simulink model "svpwm_inv_ideal_switch_Motor_new"  (R2025a)
settings: Solver=daessc  StartTime=0.0  StopTime=0.5  MaxStep=1e-7  RelTol=1e-3
undefined symbols (not defined in the file): Down, Up
libraries: fl_lib x20, nesl_utility x19, ee_lib x14, mcbeeMathTransformLib x7, slpidlib x4, eePwmGenerator x3, spsMeanLib x2, simulink_extras x1
(part 2 of 2)

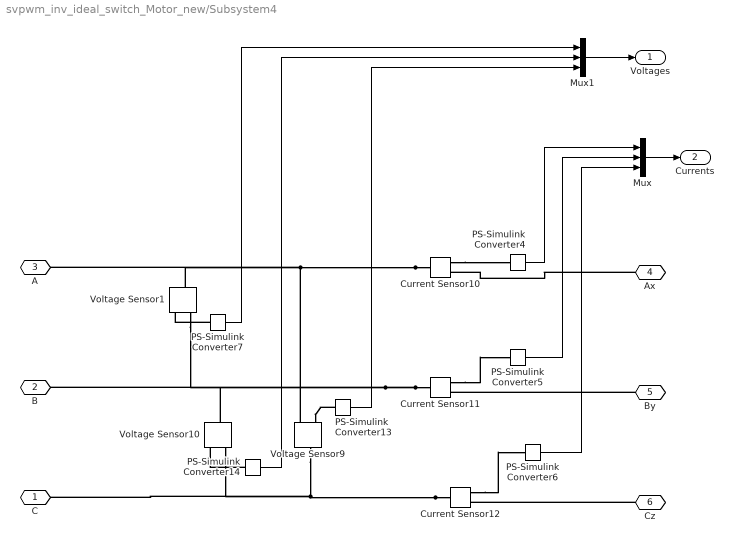
== system svpwm_inv_ideal_switch_Motor_new/Subsystem4 ==
  Current Sensor10 : fl_lib/Electrical/Electrical Sensors/Current Sensor
  Current Sensor11 : fl_lib/Electrical/Electrical Sensors/Current Sensor
  Current Sensor12 : fl_lib/Electrical/Electrical Sensors/Current Sensor
  Mux : Mux  Inputs=3
  Mux1 : Mux  Inputs=3
  PS-Simulink Converter{4..7,13..14} (6 alike) : nesl_utility/PS-Simulink Converter  PhysicalDomain=network_engine_domain  SubClassName=ps_output  LeftPortType=input  RightPortType=output  PseudoPeriodic=off  Frequencies=[]  VectorFormat=inherit  Unit=inherit  AffineConversion=off
  Voltage Sensor1 : fl_lib/Electrical/Electrical Sensors/Voltage Sensor
  Voltage Sensor10 : fl_lib/Electrical/Electrical Sensors/Voltage Sensor
  Voltage Sensor9 : fl_lib/Electrical/Electrical Sensors/Voltage Sensor
  C : PMIOPort  Side=Left
  B : PMIOPort  Port=2  Side=Left
  A : PMIOPort  Port=3  Side=Left
  Ax : PMIOPort  Port=4  Side=Right
  By : PMIOPort  Port=5  Side=Right
  Cz : PMIOPort  Port=6  Side=Right
  Voltages : Outport
  Currents : Outport  Port=2
  wires:
  Mux1/1 -> Voltages/1
  Mux/1 -> Currents/1
  PS-Simulink Converter7/1 -> Mux1/1
  PS-Simulink Converter14/1 -> Mux1/2
  PS-Simulink Converter4/1 -> Mux/1
  PS-Simulink Converter13/1 -> Mux1/3
  PS-Simulink Converter6/1 -> Mux/3
  PS-Simulink Converter5/1 -> Mux/2
  connections:
  By/RConn1 -- Current Sensor11/RConn2
  PS-Simulink Converter7/LConn1 -- Voltage Sensor1/RConn1
  PS-Simulink Converter14/LConn1 -- Voltage Sensor10/RConn1
  Current Sensor11/LConn1 -- Voltage Sensor1/RConn2 -- B/RConn1 -- Voltage Sensor10/LConn1
  Current Sensor12/RConn1 -- PS-Simulink Converter6/LConn1
  Current Sensor10/LConn1 -- Voltage Sensor9/RConn2 -- A/RConn1 -- Voltage Sensor1/LConn1
  Current Sensor12/LConn1 -- Voltage Sensor9/LConn1 -- C/RConn1 -- Voltage Sensor10/RConn2
  Current Sensor11/RConn1 -- PS-Simulink Converter5/LConn1
  Cz/RConn1 -- Current Sensor12/RConn2
  Current Sensor10/RConn1 -- PS-Simulink Converter4/LConn1
  PS-Simulink Converter13/LConn1 -- Voltage Sensor9/RConn1
  Ax/RConn1 -- Current Sensor10/RConn2

== matlab function svpwm_inv_ideal_switch_Motor_new/MATLAB Function ==
  data: a input; ag output; b input; c input; s output
function [ag,s]= fcn(a,b,c)

dt = 1/40000;
persistent Speed;
if isempty(Speed)
    Speed = 0;
end

persistent Speed_flt;
if isempty(Speed_flt)
    Speed_flt = 0;
end


persistent cnt
if isempty(cnt)
    cnt = 0;
end

persistent com_cnt
if isempty(com_cnt)
    com_cnt = 0;
end


y = a + b * 2 + c *4;
if y == 3
    ar = pi/6;
elseif y == 1
    ar = 3*pi/6;
elseif y == 5
    ar = 5*pi/6;
elseif y == 4
    ar = 7*pi/6;
elseif y == 6
    ar = 9*pi/6;
elseif y == 2
    ar = 11*pi/6;
else 
    ar = 0;
end

ar = ar-pi/6;

persistent Angle;
if isempty(Angle)
    Angle = ar;
end

if ar ~= Angle
    f = ar - Angle;
    if f<0 
        f = f + 2*pi;
    end
    Speed_new = f/dt / (cnt+1);
    if abs(Speed_new - Speed) <  max(abs(Speed*0.5),500)
        Speed = Speed_new;
    end
    cnt = 0; 
else 
    cnt = cnt + 1;
end

%if Speed > 10000
%    Speed = 0;
%end



alfa = 0.0125;

Speed_flt = Speed_flt + alfa * (Speed - Speed_flt);

Angle = ar;







if Speed_flt < 500
    ag = ar;
else 
    ag = ar + Speed_flt*dt*(cnt +1);
end

while ag > 2*pi
    ag = ag - 2*pi;
end

s = Speed_flt;
end

== matlab function svpwm_inv_ideal_switch_Motor_new/Subsystem1/SVPWM1 ==
  data: vrefa input; vphase input; VDC input; IA input; IB input; T1 output; T3 output; T5 output
function [T1, T3, T5] = fcn(vrefa,vphase, VDC, IA,IB)
%function Ts   = fcn(vrefa,vphase,VDC,IA,IB)
%время ШИМ периода
dt=50e-6;
compensate = 0;

%алгоритм формирования векторной ШИМ  мертвым веменем dead [мкс]
dead=0.0; % in us
dead_time=dead/(dt*1e6);
if (vphase < 0)
    a = vphase + 2*pi;
else
    a=vphase;
end
v2=vrefa;
if a>=0 && a<pi/3 
    n=1;
elseif  a>=pi/3 && a<2*pi/3 
    n=2;
elseif  a>=2*pi/3 && a<pi 
    n=3;
elseif  a>=pi && a<4*pi/3 
    n=4;
elseif  a>=4*pi/3 && a<5*pi/3 
    n=5;
else n=6;

end

a_cor=a-(n-1)*pi/3;

%T1 = (v2/VDC)*sin(pi/3-a_cor)/sin(pi/3);
%T2 = (v2/VDC)*sin(a_cor)/sin(pi/3);
T1 = sqrt(3) * v2/VDC *sin(pi/3 - a_cor);
T2 = sqrt(3) * v2/VDC * sin(a_cor);
T0=1-T1-T2;
Ta1=0; Ta3=0; Ta5=0; 
switch n
    case 1
        
        Ta1=T1+T2+T0/2;
        
        Ta3=T2+T0/2;
       
        Ta5=T0/2;
       
    case 2
        
        Ta1=T1+T0/2;
        
        Ta3=T1+T2+T0/2;
    
        Ta5=T0/2;       
        
    case 3
        
        Ta1=T0/2;
       
        Ta3=T1+T2+T0/2;
       
        Ta5=T2+T0/2;    
        
    case 4
        
        Ta1=T0/2;
       
        Ta3=T1+T0/2;
       
        Ta5=T1+T2+T0/2;   
       
    case 5
        
        Ta1=T2+T0/2;
        
        Ta3=T0/2;
        
        Ta5=T1+T2+T0/2;     
        
    case 6
        
        Ta1=T1+T2+T0/2;
        
        Ta3=T0/2;
     
        Ta5=T1+T0/2;    
        
end

if (Ta1 >0.995)
    Ta1 = 0.995;
elseif (Ta1 < 0.005)
        Ta1 = 0.005;
end

if (Ta3 >0.995)
    Ta3 = 0.995;
elseif (Ta3 < 0.005)
        Ta3 = 0.005;
end

if (Ta5 >0.995)
    Ta5 = 0.995;
elseif (Ta5 < 0.005)
        Ta5 = 0.005;
end

persistent start_delay;
if isempty(start_delay)
    start_delay =0;
end

if start_delay > 10
    T1 = Ta1;
    T3 = Ta3;
    T5 = Ta5;
else
    T1 = 0.5;
    T3 = 0.5;
    T5 = 0.5;
    start_delay = start_delay + 1;
end





if compensate == 1
    if (IA > 0) 
        T1 = T1 - dead_time/2;
        
    else
        T1 = T1 + dead_time/2;
         
    end

    if (IB > 0) 
        T3 = T3 - dead_time/2;

    else
        T3 = T3 + dead_time/2;

    end

    if (-(IA+IB) > 0) 
        T5 = T5 - dead_time/2;

    else
        T5 = T5 + dead_time/2;
          
    end
end


return;
